simulink model "pendulumSIM"  (R2023a)
settings: Solver=ode4  StartTime=0.0  StopTime=10  FixedStep=0.01  MaxStep=0.05  RelTol=1e-3  EnableMultiTasking=on
values from neighbouring files (symbols this model uses):
  b = 0.003    [setup_simple_pendulum.m]
  g = 9.81    [setup_simple_pendulum.m]
  IO = M * l^2    (= 0.070262)    [setup_simple_pendulum.m]
  lG = l    (= 0.43)    [setup_simple_pendulum.m]
  M = 0.380    (= 0.38)    [setup_simple_pendulum.m]
  m = 0.095    [setup_simple_pendulum.m]
  theta_dot_ic = 0    [setup_simple_pendulum.m]
  theta_ic = 0.423    [setup_simple_pendulum.m]
settings Model: Creator=richard.hill  LastModifiedBy=Fasih
settings SolverCC: AlgebraicLoopSolver=TrustRegion
settings DataIOCC: LimitDataPoints=on  ReturnWorkspaceOutputs=off
settings OptimizationCC: LifeSpan=inf
settings DebuggingCC: UnderspecifiedInitializationDetection=Classic  MergeDetectMultiDrivingBlocksExec=none  SolverPrmCheckMsg=warning  UnconnectedInputMsg=warning  UnconnectedOutputMsg=warning  UnconnectedLineMsg=warning  SFUnexpectedBacktrackingDiag=warning  SFNoUnconditionalDefaultTransitionDiag=warning  SFExecutionAtInitializationDiag=none  ArithmeticOperatorsInVariantConditions=warning
settings HardwareCC: ProdBitPerPointer=32  ProdBitPerSizeT=32  ProdBitPerPtrDiffT=32  ProdLargestAtomicFloat=None  ProdIntDivRoundTo=Undefined  ProdEndianess=Unspecified  ProdWordSize=32  ProdHWDeviceType=32-bit Generic
settings ModelReferenceCC: PropagateSignalLabelsOutOfModel=off
settings SFSimCC: SimUseLocalCustomCode=off  CustomCodeUndefinedFunction=UseInterfaceOnly
settings RTWCC: RTWUseLocalCustomCode=off
settings CodeAppCC: StateflowObjectComments=on
settings GRTTargetCC: TargetLangStandard=C89/C90 (ANSI)
settings ConfigComp: CovMetricSettings=dw  CovSaveCumulativeToWorkspaceVar=on  CovSaveSingleToWorkspaceVar=on  CovExternalEMLEnable=off

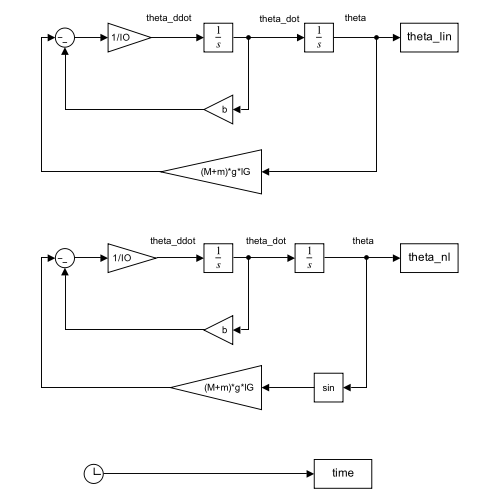
[thumbnail: Simulink's stored preview of the top-level diagram]
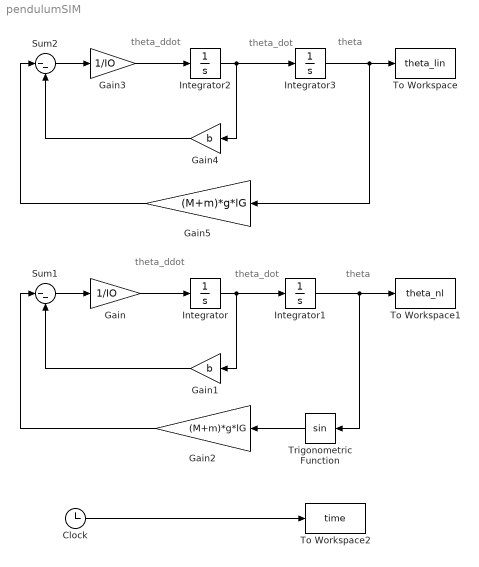
== system pendulumSIM ==
  note: theta
  note: theta_dot
  note: theta_ddot
  note: theta
  note: theta_dot
  note: theta_ddot
  Clock : Clock
  Gain : Gain  Gain=1/IO
  Gain1 : Gain  Gain=b
  Gain2 : Gain  Gain=(M+m)*g*lG
  Gain3 : Gain  Gain=1/IO
  Gain4 : Gain  Gain=b
  Gain5 : Gain  Gain=(M+m)*g*lG
  Integrator : Integrator  InitialCondition=theta_dot_ic
  Integrator1 : Integrator  InitialCondition=theta_ic
  Integrator2 : Integrator  InitialCondition=theta_dot_ic
  Integrator3 : Integrator  InitialCondition=theta_ic
  Sum1 : Sum  Inputs=|--
  Sum2 : Sum  Inputs=|--
  To Workspace : ToWorkspace  VariableName=theta_lin  SampleTime=-1
  To Workspace1 : ToWorkspace  VariableName=theta_nl  SampleTime=-1
  To Workspace2 : ToWorkspace  VariableName=time  SampleTime=-1
  Trigonometric Function : Trigonometry
  wires:
  Sum1/1 -> Gain/1
  Gain/1 -> Integrator/1
  Integrator/1 -> Gain1/1, Integrator1/1
  Integrator1/1 -> Trigonometric Function/1, To Workspace1/1
  Gain1/1 -> Sum1/2
  Trigonometric Function/1 -> Gain2/1
  Sum2/1 -> Gain3/1
  Gain3/1 -> Integrator2/1
  Integrator2/1 -> Gain4/1, Integrator3/1
  Gain4/1 -> Sum2/2
  Integrator3/1 -> Gain5/1, To Workspace/1
  Gain5/1 -> Sum2/1
  Gain2/1 -> Sum1/1
  Clock/1 -> To Workspace2/1
